simulink model "AMZ_HVPCB"  (R2022a)
settings: Solver=VariableStepAuto  StartTime=0.0  StopTime=10.0  RelTol=1e-3
undefined symbols (not defined in the file): HV_ENRE_In_Minus, HV_ENRE_In_Plus, HV_ENRE_Out_Minus, HV_ENRE_Out_Plus, HVSC_LV_In_Minus, HVSC_LV_In_Plus, HVSC_Out_Minus, HVSC_Out_Plus, LV_Minus, LV_Plus
libraries: fl_lib x15, nesl_utility x15
settings Model: Creator=joel  LastModifiedBy=sarpsepici

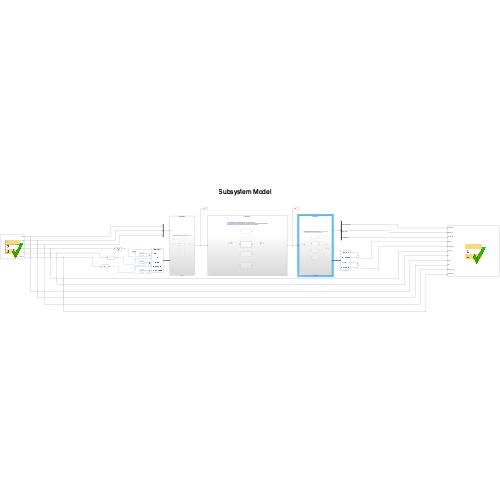
[thumbnail: Simulink's stored preview of the top-level diagram]
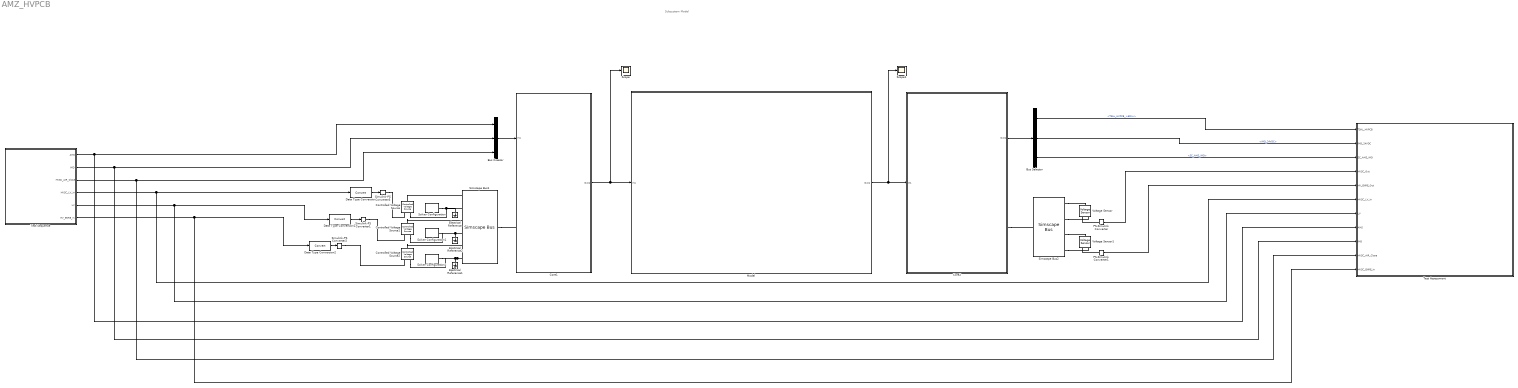
== system AMZ_HVPCB ==
  note: Subsystem Model
  Bus Creator : BusCreator  Inputs=3
  Bus Selector : BusSelector  OutputSignals=TSAL_HVPCB_>60V+,IMD_24VDC,SC_AMS_IMD
  Controlled Voltage Source : fl_lib/Electrical/Electrical Sources/Controlled Voltage Source
      settings: SourceProductBaseCode=PW,SS,VE
  Controlled Voltage Source1 : fl_lib/Electrical/Electrical Sources/Controlled Voltage Source
      settings: SourceProductBaseCode=PW,SS,VE
  Controlled Voltage Source2 : fl_lib/Electrical/Electrical Sources/Controlled Voltage Source
      settings: SourceProductBaseCode=PW,SS,VE
  Core1 : Subsystem  Variant=on
  Core2 : Subsystem  Variant=on
  Data Type Conversion : DataTypeConversion  ConvertRealWorld=Stored Integer (SI)  SaturateOnIntegerOverflow=off  RndMeth=Floor
  Data Type Conversion1 : DataTypeConversion  ConvertRealWorld=Stored Integer (SI)  SaturateOnIntegerOverflow=off  RndMeth=Floor
  Data Type Conversion2 : DataTypeConversion  ConvertRealWorld=Stored Integer (SI)  SaturateOnIntegerOverflow=off  RndMeth=Floor
  Electrical Reference : fl_lib/Electrical/Electrical Elements/Electrical Reference
      settings: SourceProductBaseCode=PW,SS,VE
  Electrical Reference1 : fl_lib/Electrical/Electrical Elements/Electrical Reference
      settings: SourceProductBaseCode=PW,SS,VE
  Electrical Reference2 : fl_lib/Electrical/Electrical Elements/Electrical Reference
      settings: SourceProductBaseCode=PW,SS,VE
  Model : Subsystem  Variant=on
  PS-Simulink Converter : nesl_utility/PS-Simulink Converter  PhysicalDomain=network_engine_domain  SubClassName=ps_output  LeftPortType=input  RightPortType=output  PseudoPeriodic=off  Frequencies=[]  VectorFormat=inherit  Unit=inherit  AffineConversion=off
      settings: SourceProductBaseCode=SS,PW,VE
  PS-Simulink Converter1 : nesl_utility/PS-Simulink Converter  PhysicalDomain=network_engine_domain  SubClassName=ps_output  LeftPortType=input  RightPortType=output  PseudoPeriodic=off  Frequencies=[]  VectorFormat=inherit  Unit=inherit  AffineConversion=off
      settings: SourceProductBaseCode=SS,PW,VE
  Scope : Scope
  Scope1 : Scope
  Simscape Bus1 : SimscapeBus  HierarchyStrings=HVSC_LV_In_Plus;HVSC_LV_In_Minus;LV_Plus;LV_Minus;HV_ENRE_In_Plus;HV_ENRE_In_Minus
  Simscape Bus2 : SimscapeBus  HierarchyStrings=HVSC_Out_Plus;HVSC_Out_Minus;HV_ENRE_Out_Plus;HV_ENRE_Out_Minus
  Simulink-PS Converter1 : nesl_utility/Simulink-PS Converter  PhysicalDomain=network_engine_domain  SubClassName=ps_input  LeftPortType=input  RightPortType=output  PseudoPeriodic=off  Frequencies=[]  NoiseDistribution=none  NoiseParameters=[]  Unit=1  AffineConversion=off  FilteringAndDerivatives=provide  SimscapeFilterOrder=1  InputFilterTimeConstant=0.001  UdotUserProvided=0
      settings: SourceProductBaseCode=SS,PW,VE
  Simulink-PS Converter2 : nesl_utility/Simulink-PS Converter  PhysicalDomain=network_engine_domain  SubClassName=ps_input  LeftPortType=input  RightPortType=output  PseudoPeriodic=off  Frequencies=[]  NoiseDistribution=none  NoiseParameters=[]  Unit=1  AffineConversion=off  FilteringAndDerivatives=provide  SimscapeFilterOrder=1  InputFilterTimeConstant=0.001  UdotUserProvided=0
      settings: SourceProductBaseCode=SS,PW,VE
  Simulink-PS Converter3 : nesl_utility/Simulink-PS Converter  PhysicalDomain=network_engine_domain  SubClassName=ps_input  LeftPortType=input  RightPortType=output  PseudoPeriodic=off  Frequencies=[]  NoiseDistribution=none  NoiseParameters=[]  Unit=1  AffineConversion=off  FilteringAndDerivatives=provide  SimscapeFilterOrder=1  InputFilterTimeConstant=0.001  UdotUserProvided=0
      settings: SourceProductBaseCode=SS,PW,VE
  Solver Configuration : nesl_utility/Solver Configuration  PhysicalDomain=network_engine_domain  SubClassName=solver  LeftPortType=input  RightPortType=generic  Tones=[]  Harmonics=[]  SimulateNoise=off  Profile=off  UseLocalSampling=off  EnableSwitchedLinearOptims=on  FrequencyDomain=off  UseCCode=off  RelTol=0.001  AbsTol=0.001  MinStep=1e-09  ToWorkspace=off  RevertToSquareIcSolve=off  NumHomotopyIterations=100  PhasorMode=off  PhasorModeNumHarmonics=1  IndexReductionMethod=DerivativeReplacement  DoDC=off  ResidualTolerance=1e-09  UseLocalSolver=off  LocalSolverChoice=NE_BACKWARD_EULER_ADVANCER  LocalSolverSampleTime=0.001  DoFixedCost=off  MaxNonlinIter=3  MaxModeIter=2  ComputeImpulses=off  ImpulseIterations=2  LinearAlgebra=auto  LinearAlgebraNumThread=0  EquationFormulation=NE_TIME_EF  DelaysMemoryBudget=1024  AutomaticFiltering=on  FilteringTimeConstant=0.001  PartitionStorageMethod=AS_NEEDED  PartitionMemoryBudget=1024  PartitionMethod=ROBUST
      settings: SourceProductBaseCode=SS,PW,VE
  Solver Configuration1 : nesl_utility/Solver Configuration  PhysicalDomain=network_engine_domain  SubClassName=solver  LeftPortType=input  RightPortType=generic  Tones=[]  Harmonics=[]  SimulateNoise=off  Profile=off  UseLocalSampling=off  EnableSwitchedLinearOptims=on  FrequencyDomain=off  UseCCode=off  RelTol=0.001  AbsTol=0.001  MinStep=1e-09  ToWorkspace=off  RevertToSquareIcSolve=off  NumHomotopyIterations=100  PhasorMode=off  PhasorModeNumHarmonics=1  IndexReductionMethod=DerivativeReplacement  DoDC=off  ResidualTolerance=1e-09  UseLocalSolver=off  LocalSolverChoice=NE_BACKWARD_EULER_ADVANCER  LocalSolverSampleTime=0.001  DoFixedCost=off  MaxNonlinIter=3  MaxModeIter=2  ComputeImpulses=off  ImpulseIterations=2  LinearAlgebra=auto  LinearAlgebraNumThread=0  EquationFormulation=NE_TIME_EF  DelaysMemoryBudget=1024  AutomaticFiltering=on  FilteringTimeConstant=0.001  PartitionStorageMethod=AS_NEEDED  PartitionMemoryBudget=1024  PartitionMethod=ROBUST
      settings: SourceProductBaseCode=SS,PW,VE
  Solver Configuration2 : nesl_utility/Solver Configuration  PhysicalDomain=network_engine_domain  SubClassName=solver  LeftPortType=input  RightPortType=generic  Tones=[]  Harmonics=[]  SimulateNoise=off  Profile=off  UseLocalSampling=off  EnableSwitchedLinearOptims=on  FrequencyDomain=off  UseCCode=off  RelTol=0.001  AbsTol=0.001  MinStep=1e-09  ToWorkspace=off  RevertToSquareIcSolve=off  NumHomotopyIterations=100  PhasorMode=off  PhasorModeNumHarmonics=1  IndexReductionMethod=DerivativeReplacement  DoDC=off  ResidualTolerance=1e-09  UseLocalSolver=off  LocalSolverChoice=NE_BACKWARD_EULER_ADVANCER  LocalSolverSampleTime=0.001  DoFixedCost=off  MaxNonlinIter=3  MaxModeIter=2  ComputeImpulses=off  ImpulseIterations=2  LinearAlgebra=auto  LinearAlgebraNumThread=0  EquationFormulation=NE_TIME_EF  DelaysMemoryBudget=1024  AutomaticFiltering=on  FilteringTimeConstant=0.001  PartitionStorageMethod=AS_NEEDED  PartitionMemoryBudget=1024  PartitionMethod=ROBUST
      settings: SourceProductBaseCode=SS,PW,VE
  Test Assessment : Test Sequence  TreatAsAtomicUnit=on
  Test Sequence : Test Sequence  TreatAsAtomicUnit=on
  Voltage Sensor : fl_lib/Electrical/Electrical Sensors/Voltage Sensor
      settings: SourceProductBaseCode=PW,SS,VE
  Voltage Sensor1 : fl_lib/Electrical/Electrical Sensors/Voltage Sensor
      settings: SourceProductBaseCode=PW,SS,VE
  wires:
  Core1/1(Out1) -> Scope/1, Model/1(In1)
  Model/1(Out1) -> Core2/1(In1), Scope1/1
  Bus Creator/1 -> Core1/1(In1)
  Data Type Conversion/1 -> Simulink-PS Converter3/1
  Data Type Conversion1/1 -> Simulink-PS Converter1/1
  Data Type Conversion2/1 -> Simulink-PS Converter2/1
  Core2/1(Out1) -> Bus Selector/1
  Bus Selector/1 -> Test Assessment/1(TSAL_HVPCB)  "<TSAL_HVPCB_>60V+>"
  Bus Selector/2 -> Test Assessment/2(IMD_24VDC)  "<IMD_24VDC>"
  Bus Selector/3 -> Test Assessment/3(SC_AMS_IMD)  "<SC_AMS_IMD>"
  PS-Simulink Converter/1 -> Test Assessment/4(HVSC_Out)
  PS-Simulink Converter1/1 -> Test Assessment/5(HV_ENRE_Out)
  Test Sequence/4(HVSC_LV_In) -> Test Assessment/6(HVSC_LV_In), Data Type Conversion/1
  Test Sequence/5(LV) -> Test Assessment/7(LV), Data Type Conversion1/1
  Test Sequence/1(AMS) -> Test Assessment/8(AMS), Bus Creator/1
  Test Sequence/2(IMD) -> Test Assessment/9(IMD), Bus Creator/2
  Test Sequence/3(HVSC_AIR_Close) -> Test Assessment/10(HVSC_AIR_Close), Bus Creator/3
  Test Sequence/6(HV_ENRE_In) -> Test Assessment/11(HVSC_ENRE_In), Data Type Conversion2/1
  connections:
  Simscape Bus1/RConn1 -- Core1/LConn1
  Controlled Voltage Source/LConn1 -- Simscape Bus1/LConn1
  Electrical Reference/LConn1 -- Simscape Bus1/LConn2 -- Solver Configuration/RConn1 -- Controlled Voltage Source/RConn2
  Controlled Voltage Source1/LConn1 -- Simscape Bus1/LConn3
  Electrical Reference2/LConn1 -- Solver Configuration1/RConn1 -- Controlled Voltage Source1/RConn2 -- Simscape Bus1/LConn4
  Controlled Voltage Source2/LConn1 -- Simscape Bus1/LConn5
  Simscape Bus1/LConn6 -- Solver Configuration2/RConn1 -- Controlled Voltage Source2/RConn2 -- Electrical Reference1/LConn1
  Simulink-PS Converter3/RConn1 -- Controlled Voltage Source/RConn1
  Simulink-PS Converter1/RConn1 -- Controlled Voltage Source1/RConn1
  Simulink-PS Converter2/RConn1 -- Controlled Voltage Source2/RConn1
  Simscape Bus2/LConn1 -- Voltage Sensor/LConn1
  Simscape Bus2/LConn2 -- Voltage Sensor/RConn2
  PS-Simulink Converter/LConn1 -- Voltage Sensor/RConn1
  Simscape Bus2/LConn3 -- Voltage Sensor1/LConn1
  Simscape Bus2/LConn4 -- Voltage Sensor1/RConn2
  PS-Simulink Converter1/LConn1 -- Voltage Sensor1/RConn1
  Core2/RConn1 -- Simscape Bus2/RConn1

== system AMZ_HVPCB/Core1 ==
  note: 1) Add Subsystem or Model blocks as valid variant choices.
      | 2) You cannot connect blocks at this level. At simulation, connectivity is automatically
      | determined, based on the active variant and port name matching.
  In1 : Inport
  Complex Model : Subsystem  VariantControl=false
  HIL : Subsystem  VariantControl=false
  Realistic Model : Subsystem  VariantControl=false
  Simple Model : Subsystem  VariantControl=true
  Connection Port : PMIOPort  Side=Left
  Out1 : Outport

== system AMZ_HVPCB/Core2 ==
  note: 1) Add Subsystem or Model blocks as valid variant choices.
      | 2) You cannot connect blocks at this level. At simulation, connectivity is automatically
      | determined, based on the active variant and port name matching.
  In1 : Inport
  Complex Model : Subsystem  VariantControl=false
  HIL : Subsystem  VariantControl=false
  Realistic Model : Subsystem  VariantControl=false
  Simple Model : Subsystem  VariantControl=true
  Connection Port : PMIOPort  Side=Right
  Out1 : Outport

== system AMZ_HVPCB/Model ==
  note: 1) Add Subsystem or Model blocks as valid variant choices.
      | 2) You cannot connect blocks at this level. At simulation, connectivity is automatically
      | determined, based on the active variant and port name matching.
  In1 : Inport
  Complex Model : Subsystem  VariantControl=false
  HIL : Subsystem  VariantControl=false
  Realistic Model : Subsystem  VariantControl=false
  Simple Model : Subsystem  VariantControl=true
  Out1 : Outport

== system AMZ_HVPCB/Core1/Complex Model ==
  In1 : Inport
  Out1 : Outport

== system AMZ_HVPCB/Core1/HIL ==
  In1 : Inport
  Out1 : Outport

== system AMZ_HVPCB/Core1/Realistic Model ==
  In1 : Inport
  Out1 : Outport

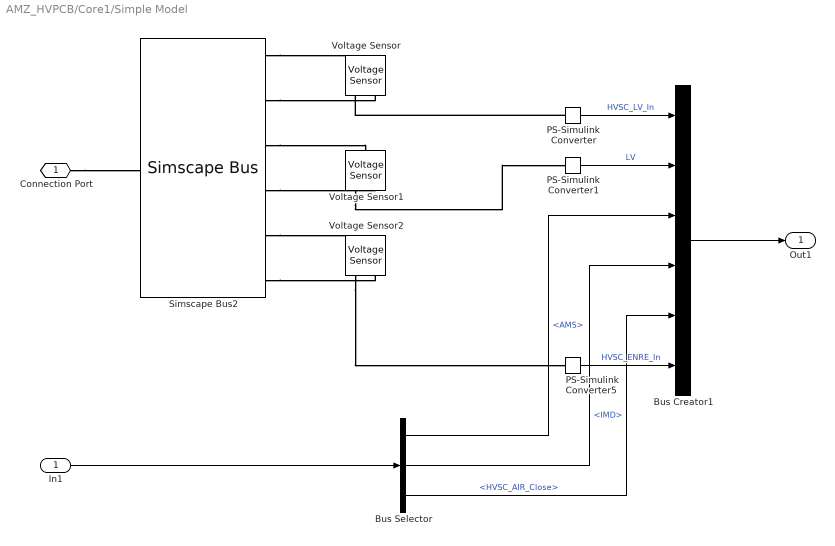
== system AMZ_HVPCB/Core1/Simple Model ==
  In1 : Inport
  Bus Creator1 : BusCreator  Inputs=6
  Bus Selector : BusSelector  OutputSignals=AMS,IMD,HVSC_AIR_Close
  PS-Simulink Converter : nesl_utility/PS-Simulink Converter  PhysicalDomain=network_engine_domain  SubClassName=ps_output  LeftPortType=input  RightPortType=output  PseudoPeriodic=off  Frequencies=[]  VectorFormat=inherit  Unit=inherit  AffineConversion=off
      settings: SourceProductBaseCode=SS,PW,VE
  PS-Simulink Converter1 : nesl_utility/PS-Simulink Converter  PhysicalDomain=network_engine_domain  SubClassName=ps_output  LeftPortType=input  RightPortType=output  PseudoPeriodic=off  Frequencies=[]  VectorFormat=inherit  Unit=inherit  AffineConversion=off
      settings: SourceProductBaseCode=SS,PW,VE
  PS-Simulink Converter5 : nesl_utility/PS-Simulink Converter  PhysicalDomain=network_engine_domain  SubClassName=ps_output  LeftPortType=input  RightPortType=output  PseudoPeriodic=off  Frequencies=[]  VectorFormat=inherit  Unit=inherit  AffineConversion=off
      settings: SourceProductBaseCode=SS,PW,VE
  Simscape Bus2 : SimscapeBus  HierarchyStrings=HVSC_LV_In_Plus;HVSC_LV_In_Minus;LV_Plus;LV_Minus;HV_ENRE_In_Plus;HV_ENRE_In_Minus
  Voltage Sensor : fl_lib/Electrical/Electrical Sensors/Voltage Sensor
      settings: SourceProductBaseCode=PW,SS,VE
  Voltage Sensor1 : fl_lib/Electrical/Electrical Sensors/Voltage Sensor
      settings: SourceProductBaseCode=PW,SS,VE
  Voltage Sensor2 : fl_lib/Electrical/Electrical Sensors/Voltage Sensor
      settings: SourceProductBaseCode=PW,SS,VE
  Connection Port : PMIOPort  Side=Left
  Out1 : Outport
  wires:
  PS-Simulink Converter/1 -> Bus Creator1/1  "HVSC_LV_In"
  PS-Simulink Converter1/1 -> Bus Creator1/2  "LV"
  Bus Creator1/1 -> Out1/1
  PS-Simulink Converter5/1 -> Bus Creator1/6  "HVSC_ENRE_In"
  In1/1 -> Bus Selector/1
  Bus Selector/1 -> Bus Creator1/3  "<AMS>"
  Bus Selector/2 -> Bus Creator1/4  "<IMD>"
  Bus Selector/3 -> Bus Creator1/5  "<HVSC_AIR_Close>"
  connections:
  Simscape Bus2/LConn1 -- Voltage Sensor/LConn1
  Simscape Bus2/LConn2 -- Voltage Sensor/RConn2
  PS-Simulink Converter/LConn1 -- Voltage Sensor/RConn1
  Simscape Bus2/LConn3 -- Voltage Sensor1/LConn1
  Simscape Bus2/LConn4 -- Voltage Sensor1/RConn2
  Simscape Bus2/LConn6 -- Voltage Sensor2/RConn2
  Voltage Sensor1/RConn1 -- PS-Simulink Converter1/LConn1
  Voltage Sensor2/RConn1 -- PS-Simulink Converter5/LConn1
  Connection Port/RConn1 -- Simscape Bus2/RConn1
  Simscape Bus2/LConn5 -- Voltage Sensor2/LConn1

== system AMZ_HVPCB/Core2/Complex Model ==
  In1 : Inport
  Out1 : Outport

== system AMZ_HVPCB/Core2/HIL ==
  In1 : Inport
  Out1 : Outport

== system AMZ_HVPCB/Core2/Realistic Model ==
  In1 : Inport
  Out1 : Outport

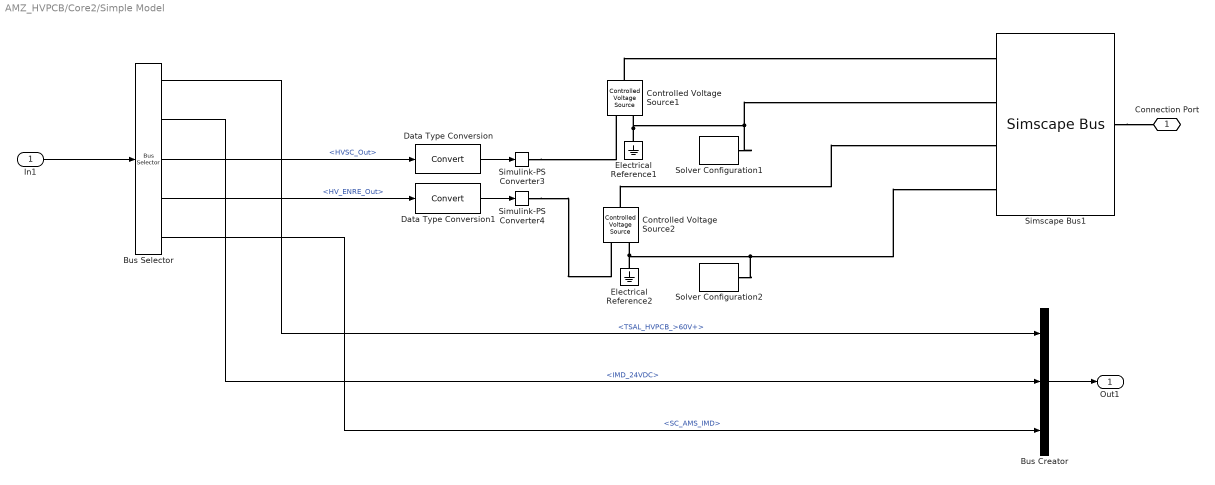
== system AMZ_HVPCB/Core2/Simple Model ==
  In1 : Inport
  Bus Creator : BusCreator  Inputs=3
  Bus Selector : BusSelector  OutputSignals=TSAL_HVPCB_>60V+,IMD_24VDC,HVSC_Out,HV_ENRE_Out,SC_AMS_IMD
  Controlled Voltage Source1 : fl_lib/Electrical/Electrical Sources/Controlled Voltage Source
      settings: SourceProductBaseCode=PW,SS,VE
  Controlled Voltage Source2 : fl_lib/Electrical/Electrical Sources/Controlled Voltage Source
      settings: SourceProductBaseCode=PW,SS,VE
  Data Type Conversion : DataTypeConversion  ConvertRealWorld=Stored Integer (SI)  SaturateOnIntegerOverflow=off  RndMeth=Floor
  Data Type Conversion1 : DataTypeConversion  ConvertRealWorld=Stored Integer (SI)  SaturateOnIntegerOverflow=off  RndMeth=Floor
  Electrical Reference1 : fl_lib/Electrical/Electrical Elements/Electrical Reference
      settings: SourceProductBaseCode=PW,SS,VE
  Electrical Reference2 : fl_lib/Electrical/Electrical Elements/Electrical Reference
      settings: SourceProductBaseCode=PW,SS,VE
  Simscape Bus1 : SimscapeBus  HierarchyStrings=HVSC_Out_Plus;HVSC_Out_Minus;HV_ENRE_Out_Plus;HV_ENRE_Out_Minus
  Simulink-PS Converter3 : nesl_utility/Simulink-PS Converter  PhysicalDomain=network_engine_domain  SubClassName=ps_input  LeftPortType=input  RightPortType=output  PseudoPeriodic=off  Frequencies=[]  NoiseDistribution=none  NoiseParameters=[]  Unit=1  AffineConversion=off  FilteringAndDerivatives=provide  SimscapeFilterOrder=1  InputFilterTimeConstant=0.001  UdotUserProvided=0
      settings: SourceProductBaseCode=SS,PW,VE
  Simulink-PS Converter4 : nesl_utility/Simulink-PS Converter  PhysicalDomain=network_engine_domain  SubClassName=ps_input  LeftPortType=input  RightPortType=output  PseudoPeriodic=off  Frequencies=[]  NoiseDistribution=none  NoiseParameters=[]  Unit=1  AffineConversion=off  FilteringAndDerivatives=provide  SimscapeFilterOrder=1  InputFilterTimeConstant=0.001  UdotUserProvided=0
      settings: SourceProductBaseCode=SS,PW,VE
  Solver Configuration1 : nesl_utility/Solver Configuration  PhysicalDomain=network_engine_domain  SubClassName=solver  LeftPortType=input  RightPortType=generic  Tones=[]  Harmonics=[]  SimulateNoise=off  Profile=off  UseLocalSampling=off  EnableSwitchedLinearOptims=on  FrequencyDomain=off  UseCCode=off  RelTol=0.001  AbsTol=0.001  MinStep=1e-09  ToWorkspace=off  RevertToSquareIcSolve=off  NumHomotopyIterations=100  PhasorMode=off  PhasorModeNumHarmonics=1  IndexReductionMethod=DerivativeReplacement  DoDC=off  ResidualTolerance=1e-09  UseLocalSolver=off  LocalSolverChoice=NE_BACKWARD_EULER_ADVANCER  LocalSolverSampleTime=0.001  DoFixedCost=off  MaxNonlinIter=3  MaxModeIter=2  ComputeImpulses=off  ImpulseIterations=2  LinearAlgebra=auto  LinearAlgebraNumThread=0  EquationFormulation=NE_TIME_EF  DelaysMemoryBudget=1024  AutomaticFiltering=on  FilteringTimeConstant=0.001  PartitionStorageMethod=AS_NEEDED  PartitionMemoryBudget=1024  PartitionMethod=ROBUST
      settings: SourceProductBaseCode=SS,PW,VE
  Solver Configuration2 : nesl_utility/Solver Configuration  PhysicalDomain=network_engine_domain  SubClassName=solver  LeftPortType=input  RightPortType=generic  Tones=[]  Harmonics=[]  SimulateNoise=off  Profile=off  UseLocalSampling=off  EnableSwitchedLinearOptims=on  FrequencyDomain=off  UseCCode=off  RelTol=0.001  AbsTol=0.001  MinStep=1e-09  ToWorkspace=off  RevertToSquareIcSolve=off  NumHomotopyIterations=100  PhasorMode=off  PhasorModeNumHarmonics=1  IndexReductionMethod=DerivativeReplacement  DoDC=off  ResidualTolerance=1e-09  UseLocalSolver=off  LocalSolverChoice=NE_BACKWARD_EULER_ADVANCER  LocalSolverSampleTime=0.001  DoFixedCost=off  MaxNonlinIter=3  MaxModeIter=2  ComputeImpulses=off  ImpulseIterations=2  LinearAlgebra=auto  LinearAlgebraNumThread=0  EquationFormulation=NE_TIME_EF  DelaysMemoryBudget=1024  AutomaticFiltering=on  FilteringTimeConstant=0.001  PartitionStorageMethod=AS_NEEDED  PartitionMemoryBudget=1024  PartitionMethod=ROBUST
      settings: SourceProductBaseCode=SS,PW,VE
  Connection Port : PMIOPort  Side=Right
  Out1 : Outport
  wires:
  In1/1 -> Bus Selector/1
  Bus Selector/1 -> Bus Creator/1  "<TSAL_HVPCB_>60V+>"
  Bus Selector/2 -> Bus Creator/2  "<IMD_24VDC>"
  Bus Selector/5 -> Bus Creator/3  "<SC_AMS_IMD>"
  Bus Creator/1 -> Out1/1
  Bus Selector/3 -> Data Type Conversion/1  "<HVSC_Out>"
  Data Type Conversion/1 -> Simulink-PS Converter3/1
  Bus Selector/4 -> Data Type Conversion1/1  "<HV_ENRE_Out>"
  Data Type Conversion1/1 -> Simulink-PS Converter4/1
  connections:
  Simulink-PS Converter3/RConn1 -- Controlled Voltage Source1/RConn1
  Simulink-PS Converter4/RConn1 -- Controlled Voltage Source2/RConn1
  Electrical Reference1/LConn1 -- Solver Configuration1/RConn1 -- Simscape Bus1/LConn2 -- Controlled Voltage Source1/RConn2
  Electrical Reference2/LConn1 -- Solver Configuration2/RConn1 -- Simscape Bus1/LConn4 -- Controlled Voltage Source2/RConn2
  Simscape Bus1/RConn1 -- Connection Port/RConn1
  Controlled Voltage Source1/LConn1 -- Simscape Bus1/LConn1
  Controlled Voltage Source2/LConn1 -- Simscape Bus1/LConn3

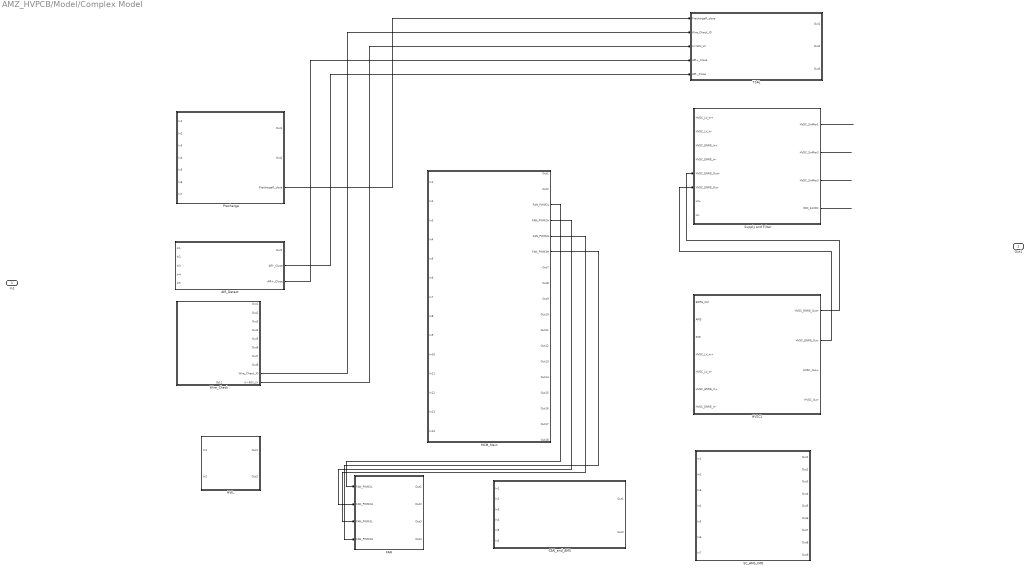
== system AMZ_HVPCB/Model/Complex Model ==
  In1 : Inport
  AIR_Detect : Subsystem
  CAN_and_AMS : Subsystem
  FAN : Subsystem
  HVIL : Subsystem
  HVSC1 : Subsystem
  MCM_Main : Subsystem
  Precharge : Subsystem
  SC_AMS_IMD : Subsystem
  Supply and Filter : Subsystem
  TSAL : Subsystem
  Wire_Check : Subsystem
      settings: PortSchema="{\"entries\":[{\"content\":{\"sides\":[{\"content\":{\"connectorIds\":[]},\"type\":\"ConnectorPlacement.EquallySpacedRectSide\",\"uuid\":\"126eba25-65f6-4658-a877-e8aa7fa1c425\"},{\"content\":{\"connectorIds\":[\"Out1\",\"Out2\",\"Out3\",\"Out4\",\"Out5\",\"Out6\",\"Out7\",\"Out8\",\"Out9\",\"Out10\"],\"side\":\"RIGHT\"},\"type\":\"ConnectorPlacement.EquallySpacedRectSide\",\"uuid\":\"4c9dfb71-69dd-4c3c-ba01-8d976b4ceda5\"},{\"content\":{\"connectorIds\":[],\"side\":\"TOP\"},\"type\":\"ConnectorPlacement.EquallySpacedRectSide\",\"uuid\":\"d5ce78f2-db3f-4ae4-a763-5d8eb57dabd0\"},{\"content\":{\"connectorIds\":[\"Out11\"],\"side\":\"BOTTOM\"},\"type\":\"ConnectorPlacement.EquallySpacedRectSide\",\"uuid\":\"e9ea3986-f9f6-4139-ba55-f695dfa270af\"}]},\"type\":\"ConnectorPlacement.EquallySpacedConnector\",\"uuid\":\"7cce0e9e-1ce4-4918-97a9-6c253ef77bbc\"}],\"packageUris\":[\"http://schema.mathworks.com/mf0/Connector/R2020b\"],\"version\":\"1.0\"}"
  Out1 : Outport
  wires:
  ? -> HVSC1/4(HVSC_LV_In+), Supply and Filter/1(HVSC_LV_In+)
  ? -> HVSC1/1(ENRE_Ctrl)
  ? -> HVSC1/3(IMD)
  Supply and Filter/3(HVSC_Sniffer3) -> ?
  ? -> HVSC1/5(HVSC_LV_In-), Supply and Filter/2(HVSC_LV_In-)
  ? -> HVSC1/7(HVSC_ENRE_In-), Supply and Filter/4(HVSC_ENRE_In-)
  AIR_Detect/3(AIR+_Close) -> TSAL/4(AIR+_Close)
  Supply and Filter/1(HVSC_Sniffer1) -> ?
  Supply and Filter/2(HVSC_Sniffer2) -> ?
  ? -> HVSC1/6(HVSC_ENRE_In+), Supply and Filter/3(HVSC_ENRE_In+)
  ? -> HVSC1/2(AMS)
  HVSC1/1(HVSC_ENRE_Out+) -> Supply and Filter/5(HVSC_ENRE_Out+)
  Supply and Filter/4(IMD_24VDC) -> ?
  AIR_Detect/2(AIR-_Close) -> TSAL/5(AIR-_Close)
  MCM_Main/4(FAN_PWM2H) -> FAN/2(FAN_PWM2H)
  Precharge/3(PrechargeR_close) -> TSAL/1(PrechargeR_close)
  HVSC1/2(HVSC_ENRE_Out-) -> Supply and Filter/6(HVSC_ENRE_Out-)
  Wire_Check/10(U>60V_LV) -> TSAL/3(U>60V_LV)
  Wire_Check/9(Wire_Check_IO) -> TSAL/2(Wire_Check_IO)
  MCM_Main/6(FAN_PWM3H) -> FAN/4(FAN_PWM3H)
  MCM_Main/5(FAN_PWM3L) -> FAN/3(FAN_PWM3L)
  MCM_Main/3(FAN_PWM2L) -> FAN/1(FAN_PWM2L)

== system AMZ_HVPCB/Model/HIL ==
  In1 : Inport
  Out1 : Outport

== system AMZ_HVPCB/Model/Realistic Model ==
  In1 : Inport
  Out1 : Outport

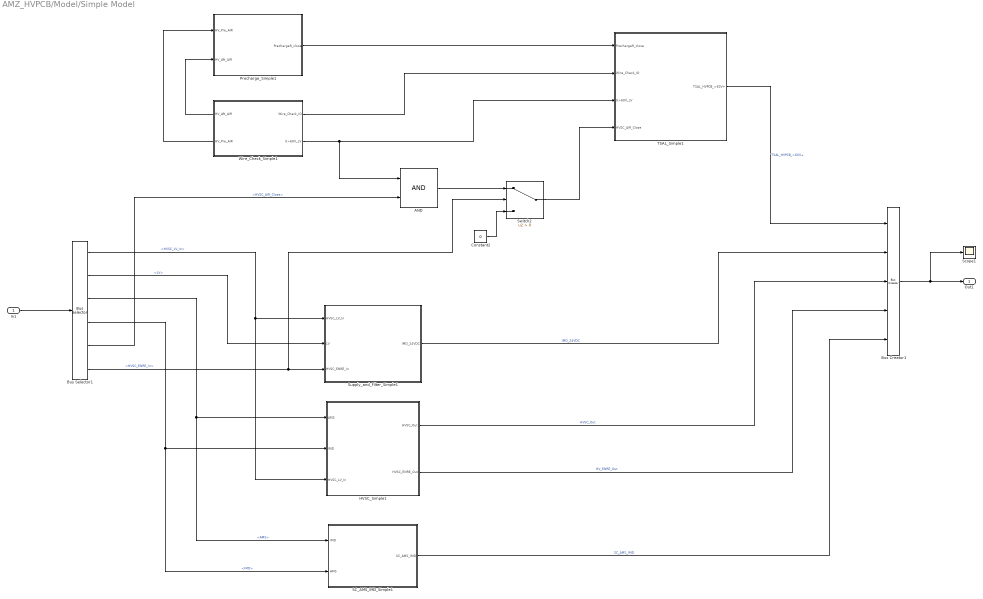
== system AMZ_HVPCB/Model/Simple Model ==
  In1 : Inport
  AND : Logic  IconShape=distinctive  AllPortsSameDT=off  OutDataTypeStr=boolean
  Bus Creator1 : BusCreator  Inputs=5
  Bus Selector1 : BusSelector  OutputSignals=HVSC_LV_In,LV,AMS,IMD,HVSC_AIR_Close,HVSC_ENRE_In
  Constant2 : Constant  Value=0  OutDataTypeStr=boolean
  HVSC_Simple1 : Subsystem
  Precharge_Simple1 : Subsystem
  SC_AMS_IMD_Simple1 : Subsystem
  Scope1 : Scope
  Supply_and_Filter_Simple1 : Subsystem
  Switch2 : Switch  Criteria=u2 > Threshold  SaturateOnIntegerOverflow=off  InputSameDT=off
  TSAL_Simple1 : Subsystem
  Wire_Check_Simple1 : Subsystem
      settings: PortSchema="{\"entries\":[{\"content\":{\"sides\":[{\"content\":{\"connectorIds\":[\"Out3\",\"Out4\"]},\"type\":\"ConnectorPlacement.EquallySpacedRectSide\",\"uuid\":\"11dacae3-814a-4f6b-acb3-fd5ffa23bd0f\"},{\"content\":{\"connectorIds\":[\"Out1\",\"Out2\"],\"side\":\"RIGHT\"},\"type\":\"ConnectorPlacement.EquallySpacedRectSide\",\"uuid\":\"4d822fac-345f-4414-ab15-0336600963b4\"},{\"content\":{\"connectorIds\":[],\"side\":\"TOP\"},\"type\":\"ConnectorPlacement.EquallySpacedRectSide\",\"uuid\":\"3e56e5dd-2c44-4fa2-bd64-4ab7ef3722be\"},{\"content\":{\"connectorIds\":[],\"side\":\"BOTTOM\"},\"type\":\"ConnectorPlacement.EquallySpacedRectSide\",\"uuid\":\"6503d3ea-34e5-4249-aa0b-a5d1e9f87ebe\"}]},\"type\":\"ConnectorPlacement.EquallySpacedConnector\",\"uuid\":\"7580b017-dc50-4084-a25b-9baedf9225fb\"}],\"packageUris\":[\"http://schema.mathworks.com/mf0/Connector/R2020b\"],\"version\":\"1.0\"}"
  Out1 : Outport
  wires:
  In1/1 -> Bus Selector1/1
  Bus Selector1/1 -> HVSC_Simple1/3(HVSC_LV_In), Supply_and_Filter_Simple1/1(HVSC_LV_In)  "<HVSC_LV_In>"
  Bus Selector1/2 -> Supply_and_Filter_Simple1/2(LV)  "<LV>"
  Bus Selector1/3 -> HVSC_Simple1/1(AMS), SC_AMS_IMD_Simple1/1(IMD)  "<AMS>"
  Bus Selector1/4 -> SC_AMS_IMD_Simple1/2(AMS), HVSC_Simple1/2(IMD)  "<IMD>"
  Bus Selector1/5 -> AND/2  "<HVSC_AIR_Close>"
  Bus Selector1/6 -> Switch2/2, Supply_and_Filter_Simple1/3(HVSC_ENRE_In)  "<HVSC_ENRE_In>"
  Wire_Check_Simple1/3(HV_Aft_AIR) -> Precharge_Simple1/2(HV_Aft_AIR)
  Wire_Check_Simple1/4(HV_Pre_AIR) -> Precharge_Simple1/1(HV_Pre_AIR)
  Precharge_Simple1/1(PrechargeR_close) -> TSAL_Simple1/1(PrechargeR_close)
  Wire_Check_Simple1/1(Wire_Check_IO) -> TSAL_Simple1/2(Wire_Check_IO)
  Wire_Check_Simple1/2(U>60V_LV) -> TSAL_Simple1/3(U>60V_LV), AND/1
  AND/1 -> Switch2/1
  Constant2/1 -> Switch2/3
  Switch2/1 -> TSAL_Simple1/4(HVSC_AIR_Close)
  TSAL_Simple1/1(TSAL_HVPCB_>60V+) -> Bus Creator1/1  "TSAL_HVPCB_>60V+"
  Supply_and_Filter_Simple1/1(IMD_24VDC) -> Bus Creator1/2  "IMD_24VDC"
  HVSC_Simple1/1(HVSC_Out) -> Bus Creator1/3  "HVSC_Out"
  HVSC_Simple1/2(HVSC_ENRE_Out) -> Bus Creator1/4  "HV_ENRE_Out"
  SC_AMS_IMD_Simple1/1(SC_AMS_IMD) -> Bus Creator1/5  "SC_AMS_IMD"
  Bus Creator1/1 -> Out1/1, Scope1/1

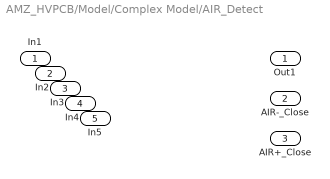
== system AMZ_HVPCB/Model/Complex Model/AIR_Detect ==
  In1 : Inport
  In2 : Inport  Port=2
  In3 : Inport  Port=3
  In4 : Inport  Port=4
  In5 : Inport  Port=5
  Out1 : Outport
  AIR-_Close : Outport  Port=2
  AIR+_Close : Outport  Port=3

== system AMZ_HVPCB/Model/Complex Model/CAN_and_AMS ==
  In1 : Inport
  In2 : Inport  Port=2
  In3 : Inport  Port=3
  In4 : Inport  Port=4
  In5 : Inport  Port=5
  In6 : Inport  Port=6
  Out1 : Outport
  Out2 : Outport  Port=2

== system AMZ_HVPCB/Model/Complex Model/FAN ==
  FAN_PWM2L : Inport
  FAN_PWM2H : Inport  Port=2
  FAN_PWM3L : Inport  Port=3
  FAN_PWM3H : Inport  Port=4
  Out1 : Outport
  Out2 : Outport  Port=2
  Out3 : Outport  Port=3
  Out4 : Outport  Port=4

== system AMZ_HVPCB/Model/Complex Model/HVIL ==
  In1 : Inport
  In2 : Inport  Port=2
  Out1 : Outport
  Out2 : Outport  Port=2

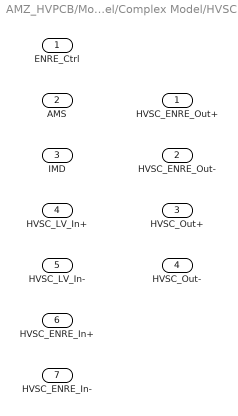
== system AMZ_HVPCB/Model/Complex Model/HVSC1 ==
  ENRE_Ctrl : Inport
  AMS : Inport  Port=2
  IMD : Inport  Port=3
  HVSC_LV_In+ : Inport  Port=4
  HVSC_LV_In- : Inport  Port=5
  HVSC_ENRE_In+ : Inport  Port=6
  HVSC_ENRE_In- : Inport  Port=7
  HVSC_ENRE_Out+ : Outport
  HVSC_ENRE_Out- : Outport  Port=2
  HVSC_Out+ : Outport  Port=3
  HVSC_Out- : Outport  Port=4

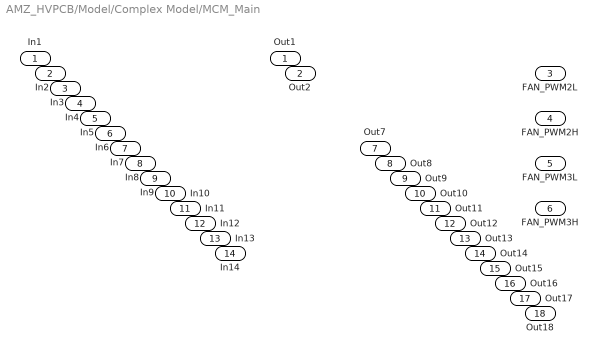
== system AMZ_HVPCB/Model/Complex Model/MCM_Main ==
  In1 : Inport
  In2 : Inport  Port=2
  In3 : Inport  Port=3
  In4 : Inport  Port=4
  In5 : Inport  Port=5
  In6 : Inport  Port=6
  In7 : Inport  Port=7
  In8 : Inport  Port=8
  In9 : Inport  Port=9
  In10 : Inport  Port=10
  In11 : Inport  Port=11
  In12 : Inport  Port=12
  In13 : Inport  Port=13
  In14 : Inport  Port=14
  Out1 : Outport
  Out2 : Outport  Port=2
  FAN_PWM2L : Outport  Port=3
  FAN_PWM2H : Outport  Port=4
  FAN_PWM3L : Outport  Port=5
  FAN_PWM3H : Outport  Port=6
  Out7 : Outport  Port=7
  Out8 : Outport  Port=8
  Out9 : Outport  Port=9
  Out10 : Outport  Port=10
  Out11 : Outport  Port=11
  Out12 : Outport  Port=12
  Out13 : Outport  Port=13
  Out14 : Outport  Port=14
  Out15 : Outport  Port=15
  Out16 : Outport  Port=16
  Out17 : Outport  Port=17
  Out18 : Outport  Port=18

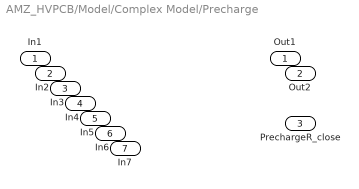
== system AMZ_HVPCB/Model/Complex Model/Precharge ==
  In1 : Inport
  In2 : Inport  Port=2
  In3 : Inport  Port=3
  In4 : Inport  Port=4
  In5 : Inport  Port=5
  In6 : Inport  Port=6
  In7 : Inport  Port=7
  Out1 : Outport
  Out2 : Outport  Port=2
  PrechargeR_close : Outport  Port=3

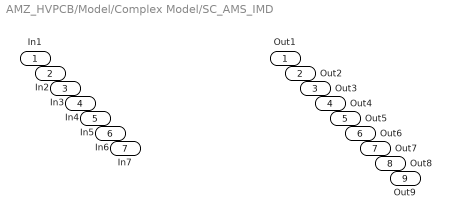
== system AMZ_HVPCB/Model/Complex Model/SC_AMS_IMD ==
  In1 : Inport
  In2 : Inport  Port=2
  In3 : Inport  Port=3
  In4 : Inport  Port=4
  In5 : Inport  Port=5
  In6 : Inport  Port=6
  In7 : Inport  Port=7
  Out1 : Outport
  Out2 : Outport  Port=2
  Out3 : Outport  Port=3
  Out4 : Outport  Port=4
  Out5 : Outport  Port=5
  Out6 : Outport  Port=6
  Out7 : Outport  Port=7
  Out8 : Outport  Port=8
  Out9 : Outport  Port=9

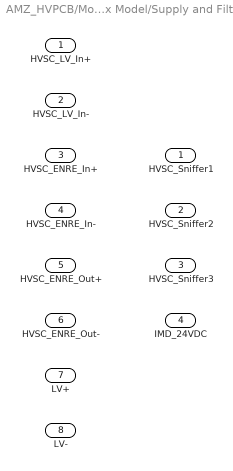
== system AMZ_HVPCB/Model/Complex Model/Supply and Filter ==
  HVSC_LV_In+ : Inport
  HVSC_LV_In- : Inport  Port=2
  HVSC_ENRE_In+ : Inport  Port=3
  HVSC_ENRE_In- : Inport  Port=4
  HVSC_ENRE_Out+ : Inport  Port=5
  HVSC_ENRE_Out- : Inport  Port=6
  LV+ : Inport  Port=7
  LV- : Inport  Port=8
  HVSC_Sniffer1 : Outport
  HVSC_Sniffer2 : Outport  Port=2
  HVSC_Sniffer3 : Outport  Port=3
  IMD_24VDC : Outport  Port=4

== system AMZ_HVPCB/Model/Complex Model/TSAL ==
  PrechargeR_close : Inport
  Wire_Check_IO : Inport  Port=2
  U>60V_LV : Inport  Port=3
  AIR+_Close : Inport  Port=4
  AIR-_Close : Inport  Port=5
  Out1 : Outport
  Out2 : Outport  Port=2
  Out3 : Outport  Port=3

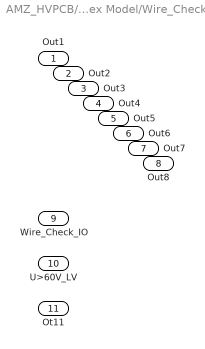
== system AMZ_HVPCB/Model/Complex Model/Wire_Check ==
  Out1 : Outport
  Out2 : Outport  Port=2
  Out3 : Outport  Port=3
  Out4 : Outport  Port=4
  Out5 : Outport  Port=5
  Out6 : Outport  Port=6
  Out7 : Outport  Port=7
  Out8 : Outport  Port=8
  Wire_Check_IO : Outport  Port=9
  U>60V_LV : Outport  Port=10
  Ot11 : Outport  Port=11

== system AMZ_HVPCB/Model/Simple Model/HVSC_Simple1 ==
  AMS : Inport
  IMD : Inport  Port=2
  HVSC_LV_In : Inport  Port=3
  AND : Logic  Inputs=3  IconShape=distinctive  AllPortsSameDT=off  OutDataTypeStr=boolean
  HVSC_Out : Outport
  HVSC_ENRE_Out : Outport  Port=2
  wires:
  AMS/1 -> AND/1
  IMD/1 -> AND/2
  HVSC_LV_In/1 -> AND/3
  AND/1 -> HVSC_ENRE_Out/1, HVSC_Out/1

== system AMZ_HVPCB/Model/Simple Model/Precharge_Simple1 ==
  HV_Pre_AIR : Inport
  HV_Aft_AIR : Inport  Port=2
  AND : Logic  IconShape=distinctive  AllPortsSameDT=off  OutDataTypeStr=boolean
  PrechargeR_close : Outport
  wires:
  HV_Pre_AIR/1 -> AND/1
  HV_Aft_AIR/1 -> AND/2
  AND/1 -> PrechargeR_close/1

== system AMZ_HVPCB/Model/Simple Model/SC_AMS_IMD_Simple1 ==
  IMD : Inport
  AMS : Inport  Port=2
  AND : Logic  IconShape=distinctive  AllPortsSameDT=off  OutDataTypeStr=boolean
  SC_AMS_IMD : Outport
  wires:
  IMD/1 -> AND/1
  AMS/1 -> AND/2
  AND/1 -> SC_AMS_IMD/1

== system AMZ_HVPCB/Model/Simple Model/Supply_and_Filter_Simple1 ==
  HVSC_LV_In : Inport
  LV : Inport  Port=2
  HVSC_ENRE_In : Inport  Port=3
  AND : Logic  Inputs=3  IconShape=distinctive  AllPortsSameDT=off  OutDataTypeStr=boolean
  IMD_24VDC : Outport
  wires:
  HVSC_LV_In/1 -> AND/1
  LV/1 -> AND/2
  AND/1 -> IMD_24VDC/1
  HVSC_ENRE_In/1 -> AND/3

== system AMZ_HVPCB/Model/Simple Model/TSAL_Simple1 ==
  PrechargeR_close : Inport
  Wire_Check_IO : Inport  Port=2
  U>60V_LV : Inport  Port=3
  HVSC_AIR_Close : Inport  Port=4
  AND : Logic  Inputs=4  IconShape=distinctive  AllPortsSameDT=off  OutDataTypeStr=boolean
  TSAL_HVPCB_>60V+ : Outport  OutDataTypeStr=boolean
  wires:
  PrechargeR_close/1 -> AND/1
  Wire_Check_IO/1 -> AND/2
  U>60V_LV/1 -> AND/3
  HVSC_AIR_Close/1 -> AND/4
  AND/1 -> TSAL_HVPCB_>60V+/1

== system AMZ_HVPCB/Model/Simple Model/Wire_Check_Simple1 ==
  Wire_Check_Boolean : Constant  OutDataTypeStr=boolean
  Wire_Check_Boolean1 : Constant  OutDataTypeStr=boolean
  Wire_Check_Boolean2 : Constant  OutDataTypeStr=boolean
  Wire_Check_IO : Outport  OutDataTypeStr=boolean
  U>60V_LV : Outport  Port=2
  HV_Aft_AIR : Outport  Port=3
  HV_Pre_AIR : Outport  Port=4
  wires:
  Wire_Check_Boolean/1 -> Wire_Check_IO/1, U>60V_LV/1
  Wire_Check_Boolean1/1 -> HV_Aft_AIR/1
  Wire_Check_Boolean2/1 -> HV_Pre_AIR/1

== stateflow chart AMZ_HVPCB/Test Sequence ==
  state step_1
    % HVSC_LV_In_Plus = 1;
    % HVSC_LV_In_Minus = 0;
    % LV_Plus = 1;
    % LV_Minus = 0;
    % HV_ENRE_In_Plus = 1;
    % HV_ENRE_In_Minus = 0;
    HVSC_LV_In = 1;
    LV = 1;
    HV_ENRE_In = 1;
    AMS = 1;
    IMD = 1;
    HVSC_AIR_Close = 1;
  state step_2
  (default) -> step_1
  step_1 -> step_2
  data: AMS output; IMD output; HVSC_AIR_Close output; HVSC_LV_In output; LV output; HV_ENRE_In output

== stateflow chart AMZ_HVPCB/Test Assessment ==
  state step_1
    state step_1_1
      % verify input values
      verify(HVSC_LV_In == 1);
      verify(LV == 1);
      verify(AMS == 1);
      verify(IMD == 1);
      verify(HVSC_AIR_Close == 1);
      verify(HVSC_ENRE_In == 1);
      % verify output values
      verify(TSAL_HVPCB == 1);
      verify(IMD_24VDC == 1);
      verify(SC_AMS_IMD == 1);
      verify(HVSC_Out == 1);
      verify(HV_ENRE_Out == 1);
      % verify HVPCB conditions
      verify(AMS & IMD & HVSC_LV_In == HVSC_Out);
      verify(AMS & IMD & HVSC_LV_In == HV_ENRE_Out);
      verify(AMS & IMD == SC_AMS_IMD);
      verify(HVSC_LV_In & LV & HVSC_ENRE_In == IMD_24VDC);
      verify(HVSC_ENRE_In & HVSC_AIR_Close == TSAL_HVPCB);
    state step_1_2
    (default) -> (junction 22)
    step_1 -> (junction 22)
    (junction 22) -> (junction 23) [order 1] : [true
        | ]
    (junction 23) -> step_1_1 [order 1] : [~in(step_1.step_1_1)]
    (junction 22) -> (junction 31) [order 2]
    (junction 23) -> (junction 26) [order 2]
    (junction 31) -> (junction 32)
    (junction 32) -> step_1_2 [order 1] : [~in(step_1.step_1_2)]
    (junction 32) -> (junction 35) [order 2]
  (default) -> step_1
  data: TSAL_HVPCB input; IMD_24VDC input; SC_AMS_IMD input; HVSC_Out input; HV_ENRE_Out input; HVSC_LV_In input; LV input; AMS input; IMD input; HVSC_AIR_Close input; HVSC_ENRE_In input
